simulink model "PVBatteryIntegrationBuck"  (R2019a)
settings: Solver=ode23t  StartTime=0.0  StopTime=1  FixedStep=10e-6  RelTol=1e-3
undefined symbols (not defined in the file or in its folder): Ion, Lithium
libraries: powerlib x6, electricdrivelib x1, re_lib x1, simulink x1
settings Model: Creator=Administrator  LastModifiedBy=Administrator

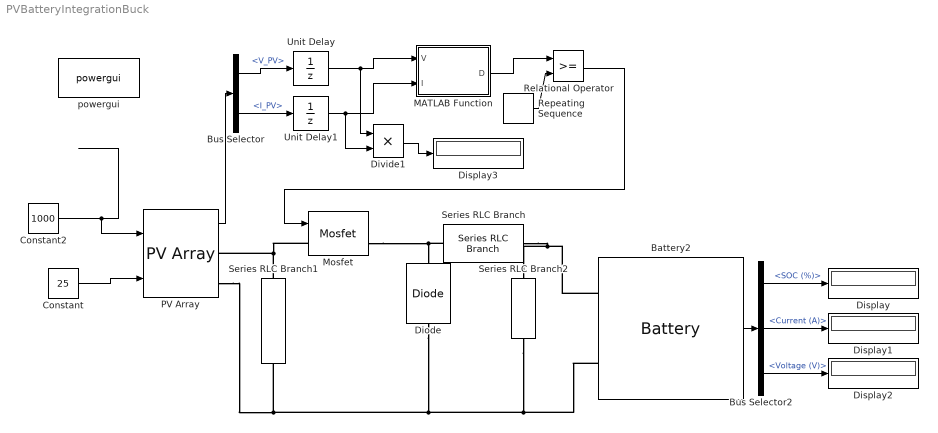
== system PVBatteryIntegrationBuck ==
  Battery2 : electricdrivelib/Extra Sources/Battery  BatType=Lithium-Ion  ShowTempParam=off  ThermalPreset=no  ShowAgeParam=off  NomV=12  NomQ=100  SOC=45  Batt_Tr=1  PresetModel=on  MaxQ=100  MinV=9  FullV=13.9678  Dis_rate=43.4783  R=0.0012  Normal_OP=90.4348  expZone="[12.9646      4.91304]"  current=[6.5 13 32.5]  Units=Time  Tci=20  NomT=20  T2=-30  MaxQ2=4.8  FullV2=7.1  Normal_OP2=5.655  expZone2="[6.58           1]"  Rca=0.6  ti=2000  Dp=0  Neq0=0  Tsim=1e6  Ta1=25  Qeol=5.4*0.9  Reol=0.013333*1.2  Char_age=[2.3478, 3]  Dis_age=[2.3478, 10]  N1=1500  N2=10500  N3=1000  N4=1400  Ta2=45  N5=950
      settings: SourceProductName=Simscape Electrical
  Bus Selector : BusSelector  OutputSignals=V_PV,I_PV
  Bus Selector2 : BusSelector  OutputSignals=SOC (%),Current (A),Voltage (V)
  Constant : Constant  Value=25
  Constant2 : Constant  Value=1000  SampleTime=10e-6
  Diode : powerlib/Power Electronics/Diode  Ron=0.001  Lon=0  Vf=0.8  IC=0  UseSnubber=0  Rs=500  Cs=250e-9  Measurements=off
      settings: SourceProductName=Simscape Electrical
  Display{,1..3} (4 alike) : Display
  Divide1 : Product  Inputs=**
  MATLAB Function : MATLAB Function  TreatAsAtomicUnit=on
  Mosfet : powerlib/Power Electronics/Mosfet  Ron=0.1  Lon=0  Rd=0.01  Vfd=0  IC=0  Rs=1e5  Cs=inf  Measurements=on
      settings: SourceProductName=Simscape Electrical
  PV Array : re_lib/Solar/PV Array  Npar=1  Nser=1  PlotType=array @ 1000 W/m2 & specified temperatures  S_vec="[ 1000  500  100 ]"  Temp_C_vec="[ 45 25  ]"  ModuleName=1Soltech 1STH-215-P  PlotWhenSelected=off  Pm=213.15  Ncell=60  Voc=36.3  Isc=7.84  Vm=29  Im=7.35  beta_Voc_pc=-0.36099  alpha_Isc_pc=0.102  beta_Voc=-0.13104  alpha_Isc=0.007997  IL=7.8649  I0=2.9259e-10  nI=0.98117  Rsh=313.3991  Rs=0.39383  BAL=on  Tc=1e-6  Tfilter=5e-5
      settings: SourceProductName=Simscape Electrical
  Relational Operator : RelationalOperator  OutDataTypeStr=boolean  RndMeth=Simplest
  Repeating Sequence : simulink/Sources/Repeating Sequence  rep_seq_t=[0 0.0002]  rep_seq_y=[0 1]
  Series RLC Branch : powerlib/Elements/Series RLC Branch  LConnTagsString=__new0  RConnTagsString=__new0  BranchType=L  Resistance=0.1  Inductance=0.783  SetiL0=off  InitialCurrent=0  Capacitance=1e-6  Setx0=off  InitialVoltage=0  Measurements=None
      settings: SourceProductName=Simscape Electrical
  Series RLC Branch1 : powerlib/Elements/Series RLC Branch  LConnTagsString=__new0  RConnTagsString=__new0  BranchType=RC  Resistance=0.0001  Inductance=1e-3  SetiL0=off  InitialCurrent=0  Capacitance=1000e-6  Setx0=off  InitialVoltage=0  Measurements=None
      settings: SourceProductName=Simscape Electrical
  Series RLC Branch2 : powerlib/Elements/Series RLC Branch  LConnTagsString=__new0  RConnTagsString=__new0  BranchType=C  Resistance=1e-4  Inductance=1e-3  SetiL0=off  InitialCurrent=0  Capacitance=364e-6  Setx0=off  InitialVoltage=0  Measurements=None
      settings: SourceProductName=Simscape Electrical
  Unit Delay : UnitDelay  SampleTime=-1  HasFrameUpgradeWarning=on
  Unit Delay1 : UnitDelay  SampleTime=-1  HasFrameUpgradeWarning=on
  powergui : powerlib/powergui  Priority=1  SimulationMode=Discrete  SampleTime=1e-6  frequency=60  Iterations=50  frequencyindice=0  Pbase=100e6  ErrMax=1e-4  UnitsV=kV  UnitsW=MW  buscounter=0  FunctionMessages=off  echomessages=off  EnableUseOfTLC=off  CurrentSourceSwitches=off  DisableSnubberDevices=off  DisableRonSwitches=off  DisableVfSwitches=off  DisplayEquations=off  AutomaticDiscreteSolvers=off  SolverType=Tustin/Backward Euler (TBE)  Interpol=off  ExternalGateDelay=off  methode=off  Ts=100  x0status=blocks  SPID=on  SwTol=0  HookPort=off  NonlinearTolerance=0  nMaxIteration=15  ContinueOnMaxIteration=off  RestoreLinks=warning  ResistiveCurrentMeasurement=off  Frange=[0:2:500]  Ylog=off  Xlog=on  ShowGrid=off  save=off  variable=ZData  structure=0  ZoomFFT=off  StartTime=0.0  cycles=1  DisplayStyle=1  fundamental=60  FreqAxis=off  MaxFrequency=1000  frequencyindicesteady=1  RmsSteady=1  display=off
      settings: SourceProductName=Simscape Electrical
  wires:
  Constant2/1 -> PV Array/1
  Bus Selector/2 -> Unit Delay1/1  "<I_PV>"
  Constant/1 -> PV Array/2
  PV Array/1 -> Bus Selector/1
  Bus Selector2/1 -> Display/1  "<SOC (%)>"
  Battery2/1 -> Bus Selector2/1
  Bus Selector2/2 -> Display1/1  "<Current (A)>"
  Bus Selector2/3 -> Display2/1  "<Voltage (V)>"
  Bus Selector/1 -> Unit Delay/1  "<V_PV>"
  Unit Delay/1 -> Divide1/1, MATLAB Function/1(V)
  Unit Delay1/1 -> Divide1/2, MATLAB Function/2(I)
  MATLAB Function/1(D) -> Relational Operator/1
  Repeating Sequence/1 -> Relational Operator/2
  Relational Operator/1 -> Mosfet/1
  Divide1/1 -> Display3/1
  connections:
  Series RLC Branch2/RConn1 -- Battery2/LConn2 -- Diode/LConn1 -- Series RLC Branch1/RConn1 -- PV Array/RConn2
  Series RLC Branch1/LConn1 -- PV Array/RConn1 -- Mosfet/LConn1
  Series RLC Branch/RConn1 -- Series RLC Branch2/LConn1 -- Battery2/LConn1
  Mosfet/RConn1 -- Series RLC Branch/LConn1 -- Diode/RConn1

== matlab function PVBatteryIntegrationBuck/MATLAB Function ==
  data: V input; D output; I input
function D=dutyRatio(V,I)
Dmax=0.95;
Dmin=0;
Dinit=0.95;
deltaD=0.0001;
persistent Vold Pold Dold;
if isempty(Vold)
    Vold=0;
    Pold=0;
    Dold=Dinit;
end
P=V*I;
dV=V-Vold;
dP=P-Pold;
if dP~=0
    if dP<0
         if dV<0
            D=Dold-deltaD;
         else
            D=Dold+deltaD;
         end
    else
         if dV<0
            D=Dold+deltaD;
         else
            D=Dold-deltaD;
         end
    end
else
    D=Dold;
end
    if D>=Dmax ||D<=Dmin
            D=Dold;
    end
            Dold=D;
            Vold=V;
            Pold=P;
